simulink model "mcb_host_model_f28069m"  (R2023b)
settings: Solver=FixedStepDiscrete  StartTime=0.0  StopTime=inf  RelTol=1e-3  EnableMultiTasking=on
values from neighbouring files (symbols this model uses):
  inverter = mcb_SetInverterParameters('SBLMB500')    [mcb_bldc_sixstep_f28069mLaunchPad_data.m]
  PU_System = mcb_SetPUSystem(bldc,inverter)    [mcb_bldc_sixstep_f28069mLaunchPad_data.m]
  Ts = 0.03    [dataMonitoringArr.m]    (also in mcb_bldc_sixstep_f28069mLaunchPad_data.m = 5e-05)
libraries: instrumentseriallib x3, dspstat3 x1
settings Model: Creator=The MathWorks, Inc.  LastModifiedBy=Tefilus
settings SolverCC: AlgebraicLoopSolver=TrustRegion  AutoInsertRateTranBlk=on  MaxZcPerStep=1
settings DataIOCC: LimitDataPoints=on  ReturnWorkspaceOutputs=off
settings OptimizationCC: ReuseModelBlockBuffer=off  LifeSpan=1  EfficientTunableParamExpr=on
settings DebuggingCC: UnderspecifiedInitializationDetection=Classic  MergeDetectMultiDrivingBlocksExec=none  SolverPrmCheckMsg=warning  ParameterPrecisionLossMsg=none  UnconnectedInputMsg=warning  UnconnectedOutputMsg=warning  UnconnectedLineMsg=warning  AllowSymbolicDim=off  PregeneratedLibrarySubsystemCodeDiagnostic=none  SFUnexpectedBacktrackingDiag=warning  SFNoUnconditionalDefaultTransitionDiag=warning  SFExecutionAtInitializationDiag=none  ArithmeticOperatorsInVariantConditions=warning
settings HardwareCC: ProdBitPerPointer=32  ProdLargestAtomicFloat=None  ProdIntDivRoundTo=Undefined  ProdEndianess=Unspecified  ProdWordSize=32  ProdHWDeviceType=32-bit Generic
settings ModelReferenceCC: EnableRefExpFcnMdlSchedulingChecks=on  PropagateSignalLabelsOutOfModel=off
settings SFSimCC: SimUseLocalCustomCode=off
settings RTWCC: Description=Real-Time Workshop Embedded Coder  SystemTargetFile=ert.tlc  TemplateMakefile=ert_default_tmf  GenerateReport=on  RTWUseLocalCustomCode=off  IncludeHyperlinkInReport=on  LaunchReport=on  GenerateTraceInfo=on  GenerateTraceReport=on  GenerateTraceReportSl=on  GenerateTraceReportSf=on  GenerateTraceReportEml=on  DLArmComputeVersion=19.05
settings CodeAppCC: IgnoreCustomStorageClasses=off  StateflowObjectComments=on  InternalIdentifier=Classic
settings ERTTargetCC: MultiwordLength=2048  GenerateSampleERTMain=on  ERTCustomFileTemplate=example_file_process.tlc  ConvertIfToSwitch=off  SuppressUnreachableDefaultCases=off
settings ConfigComp: CovMetricSettings=dw  CovSaveCumulativeToWorkspaceVar=on  CovSaveSingleToWorkspaceVar=on  CovExternalEMLEnable=off  CovSFcnEnable=off

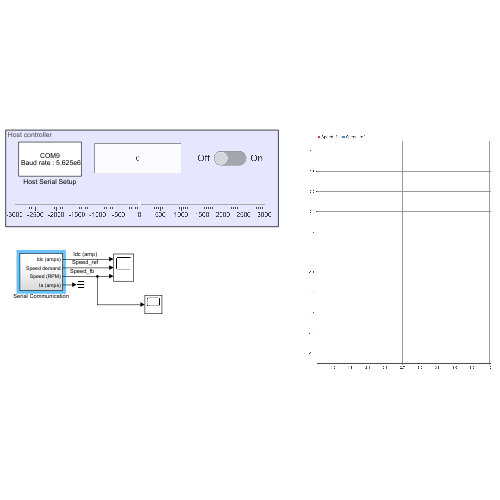
[thumbnail: Simulink's stored preview of the top-level diagram]
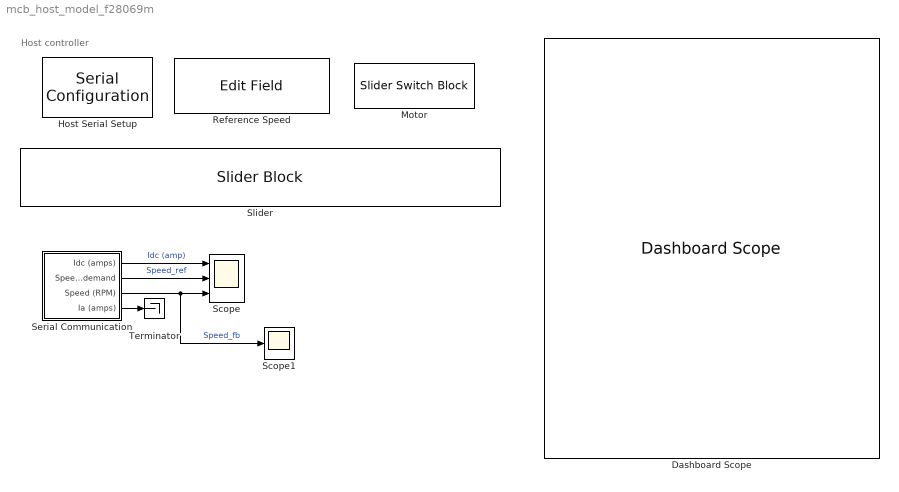
== system mcb_host_model_f28069m ==
  note: Host controller
  Dashboard Scope : DashboardScope  TimeSpan=3  Ymin=-3000  Ymax=3000  UpdateMode=Scroll
  Host Serial Setup : instrumentseriallib/Serial Configuration  Priority=-99  PortSel=target.comport  Port=target.comport  ComPort=target.comport  BaudRate=5.625e6  DataBits=8  Parity=none  StopBits=1  ByteOrder=little-endian  FlowControl=none  Timeout=2  SimulateUsing=Interpreted execution  BlockInModel=on  aMode=5
  Motor : SliderSwitchBlock  LabelPosition=Hide
      settings: Values={{'Off', 'On'}, [0 1]}
  Reference Speed : EditField  LabelPosition=Hide  ShowInitialText=on  Alignment=Center
  Scope : Scope  NumInputPorts=3
  Scope1 : Scope
  Serial Communication : Subsystem
  Slider : SliderBlock  LabelPosition=Hide  ScaleMin=-3000  ScaleMax=3000
  Terminator : Terminator
  wires:
  Serial Communication/4(Ia (amps)) -> Terminator/1
  Serial Communication/1(Idc (amps)) -> Scope/1  "Idc (amp)"
  Serial Communication/2(Speed demand) -> Scope/2  "Speed_ref"
  Serial Communication/3(Speed (RPM)) -> Scope1/1, Scope/3  "Speed_fb"

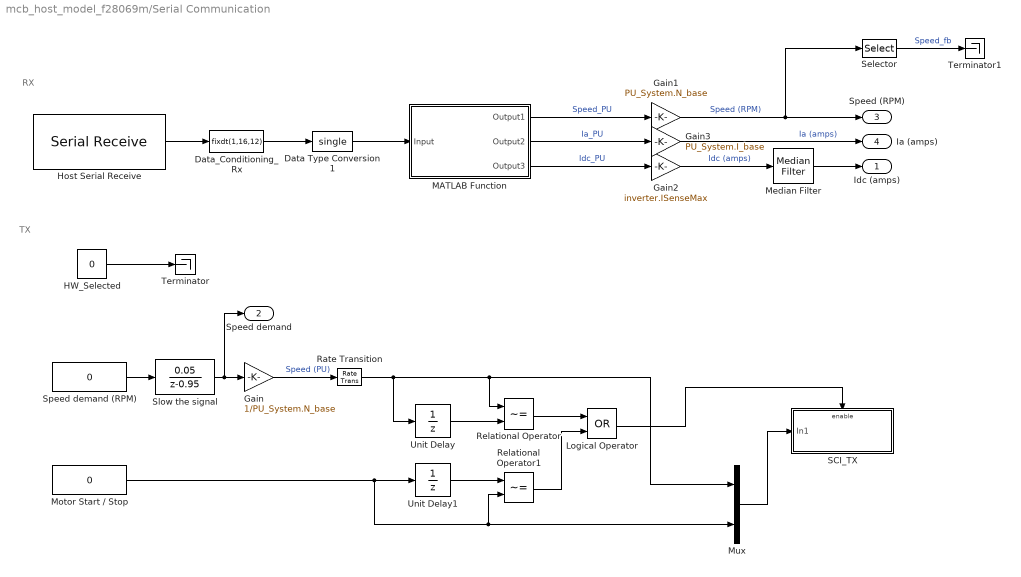
== system mcb_host_model_f28069m/Serial Communication ==
  note: RX
  note: TX
  Data Type Conversion1 : DataTypeConversion  OutDataTypeStr=single  RndMeth=Simplest  SaturateOnIntegerOverflow=off
  Data_Conditioning_Rx : DataTypeConversion  OutDataTypeStr=fixdt(1,16,12)  ConvertRealWorld=Stored Integer (SI)  RndMeth=Simplest  SaturateOnIntegerOverflow=off
  Gain : Gain  Gain=1/PU_System.N_base  RndMeth=Simplest  OutDataTypeStr=Inherit: Same as input
  Gain1 : Gain  Gain=PU_System.N_base  OutDataTypeStr=single  RndMeth=Simplest
  Gain2 : Gain  Gain=inverter.ISenseMax  OutDataTypeStr=single  RndMeth=Simplest
  Gain3 : Gain  Gain=PU_System.I_base  OutDataTypeStr=single  RndMeth=Simplest
  HW_Selected : Constant  Value=0  OutDataTypeStr=uint8
  Host Serial Receive : instrumentseriallib/Serial Receive  PortSel=target.comport  Port=target.comport  ComPort=target.comport  DataType=uint16  SaveDataType=uint8  ToggleHeader=on  Header='SS'  ToggleTerminator=on  Terminator=Custom terminator  CustomTerminator='EE'  InputFormat=Row major  ToggleDataSize=on  DataSize=[600 3]  EnableBlockingMode=on  ActionDataUnavailable=Output last received value  ActionWhenDataUnavailable=Output last received value  CustomValue=0  SampleTime=600 * Ts  SimulateUsing=Interpreted execution  BlockInModel=on  aMode=5
  Logical Operator : Logic  Operator=OR  AllPortsSameDT=off  OutDataTypeStr=boolean
  MATLAB Function : MATLAB Function  TreatAsAtomicUnit=on
  Median Filter : dspstat3/Median Filter  WindowLength=1000  SimulateUsing=Interpreted execution
      settings: LibrarySourceBlock=|
      | dspfdesign/Median
      | Filter
  Motor Start / Stop : Constant  Value=0  VectorParams1D=off  OutDataTypeStr=single  SampleTime=0.03
  Mux : Mux  Inputs=2
  Rate Transition : RateTransition  OutPortSampleTime=0.03
  Relational Operator : RelationalOperator  Operator=~=  OutDataTypeStr=boolean  InputSameDT=off
  Relational Operator1 : RelationalOperator  Operator=~=  OutDataTypeStr=boolean  InputSameDT=off
  SCI_TX : Subsystem  TreatAsAtomicUnit=on
  Selector : Selector  InputPortWidth=600  IndexOptions=Index vector (dialog)  Indices=599  OutputSizes=1
  Slow the signal : DiscreteTransferFcn  Numerator=[0.05]  Denominator=[1 -0.95]
  Speed demand (RPM) : Constant  Value=0  VectorParams1D=off  OutDataTypeStr=single  SampleTime=0.03
  Terminator : Terminator
  Terminator1 : Terminator
  Unit Delay : UnitDelay  InitialCondition=0.5  SampleTime=-1  HasFrameUpgradeWarning=on
  Unit Delay1 : UnitDelay  SampleTime=-1  HasFrameUpgradeWarning=on
  Idc (amps) : Outport
  Speed demand : Outport  Port=2
  Speed (RPM) : Outport  Port=3
  Ia (amps) : Outport  Port=4
  wires:
  HW_Selected/1 -> Terminator/1
  Unit Delay1/1 -> Relational Operator1/1
  Relational Operator1/1 -> Logical Operator/2
  Unit Delay/1 -> Relational Operator/2
  Relational Operator/1 -> Logical Operator/1
  Gain/1 -> Rate Transition/1  "Speed (PU)"
  Mux/1 -> SCI_TX/1(In1)
  Rate Transition/1 -> Unit Delay/1, Mux/1, Relational Operator/1
  Logical Operator/1 -> SCI_TX/Enable
  Motor Start / Stop/1 -> Relational Operator1/2, Mux/2, Unit Delay1/1
  MATLAB Function/2(Output2) -> Gain3/1  "Ia_PU"
  Gain3/1 -> Ia (amps)/1  "Ia (amps)"
  Host Serial Receive/1 -> Data_Conditioning_Rx/1
  MATLAB Function/1(Output1) -> Gain1/1  "Speed_PU"
  Gain1/1 -> Selector/1, Speed (RPM)/1  "Speed (RPM)"
  Data_Conditioning_Rx/1 -> Data Type Conversion1/1
  Data Type Conversion1/1 -> MATLAB Function/1(Input)
  MATLAB Function/3(Output3) -> Gain2/1  "Idc_PU"
  Median Filter/1 -> Idc (amps)/1
  Gain2/1 -> Median Filter/1  "Idc (amps)"
  Slow the signal/1 -> Speed demand/1, Gain/1
  Selector/1 -> Terminator1/1  "Speed_fb"
  Speed demand (RPM)/1 -> Slow the signal/1

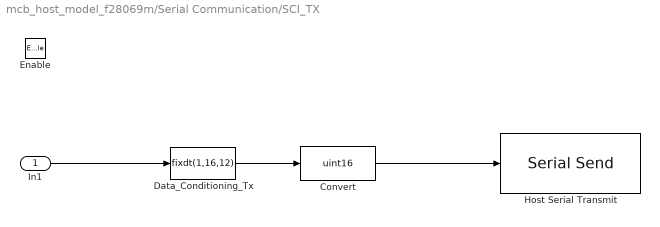
== system mcb_host_model_f28069m/Serial Communication/SCI_TX ==
  In1 : Inport
  Enable : EnablePort
  Convert : DataTypeConversion  OutDataTypeStr=uint16  ConvertRealWorld=Stored Integer (SI)  RndMeth=Simplest  SaturateOnIntegerOverflow=off
  Data_Conditioning_Tx : DataTypeConversion  OutDataTypeStr=fixdt(1,16,12)  RndMeth=Simplest  SaturateOnIntegerOverflow=off
  Host Serial Transmit : instrumentseriallib/Serial Send  PortSel=target.comport  Port=target.comport  ComPort=target.comport  Header=[]  Terminator=<none>  CustomTerminator=[]  EnableBlockingMode=off  SimulateUsing=Interpreted execution  BlockInModel=on  aMode=5
  wires:
  Convert/1 -> Host Serial Transmit/1
  Data_Conditioning_Tx/1 -> Convert/1
  In1/1 -> Data_Conditioning_Tx/1

== matlab function mcb_host_model_f28069m/Serial Communication/MATLAB Function ==
  data: Output1 output; Output2 output; Input input; Output3 output
function [ Output1, Output2, Output3] = unBuf(Input)

Output1 = Input(:, 1);
Output2 = Input(:, 2);
Output3 = Input(:, 3);
% Output4 = Input(:, 4);
end
